simulink model "Control_config"  (R2023b)
settings: Solver=VariableStepAuto  StartTime=0.0  StopTime=inf  RelTol=1e-3
libraries: vrlib x1
settings Model: Creator=angel  LastModifiedBy=angel

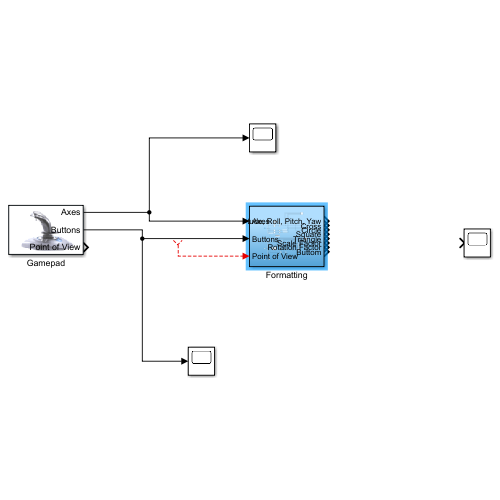
[thumbnail: Simulink's stored preview of the top-level diagram]
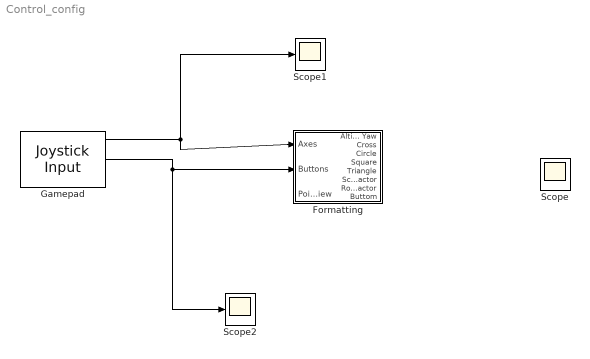
== system Control_config ==
  Formatting : Subsystem
  Gamepad : vrlib/Joystick Input  joyid=1  adjustports=on  forcefeed=off
  Scope : Scope
  Scope1 : Scope
  Scope2 : Scope
  wires:
  Gamepad/2 -> Scope2/1, Formatting/2(Buttons)
  ? -> Formatting/3(Point of View)
  Gamepad/1 -> Scope1/1, Formatting/1(Axes)

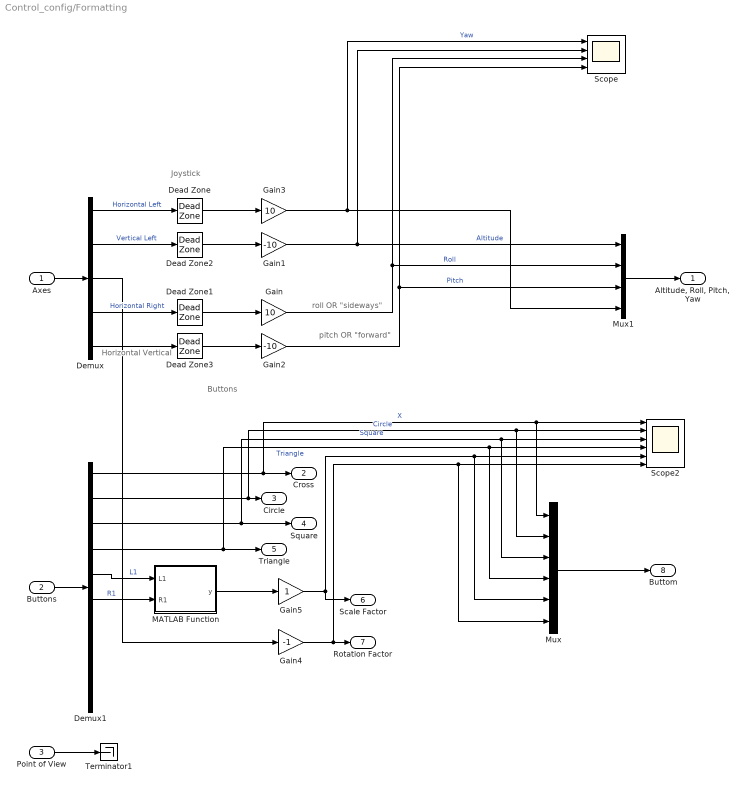
== system Control_config/Formatting ==
  note: Joystick
  note: Horizontal Vertical
  note: roll OR "sideways"
  note: pitch OR "forward"
  note: Buttons
  Axes : Inport
  Buttons : Inport  Port=2
  Point of View : Inport  Port=3
  Dead Zone{,1..3} (4 alike) : DeadZone  LowerValue=-0.2  UpperValue=0.2
  Demux : Demux  Outputs=5
  Demux1 : Demux  Outputs=10
  Gain : Gain  Gain=10
  Gain1 : Gain  Gain=-10
  Gain2 : Gain  Gain=-10
  Gain3 : Gain  Gain=10
  Gain4 : Gain  Gain=-1
  Gain5 : Gain
  MATLAB Function : MATLAB Function  TreatAsAtomicUnit=on
  Mux : Mux  Inputs=6
  Mux1 : Mux
  Scope : Scope  NumInputPorts=4
  Scope2 : Scope  NumInputPorts=6
  Terminator1 : Terminator
  "Altitude, Roll, Pitch, Yaw" : Outport
  Cross : Outport  Port=2
  Circle : Outport  Port=3
  Square : Outport  Port=4
  Triangle : Outport  Port=5
  Scale Factor : Outport  Port=6
  Rotation Factor : Outport  Port=7
  Buttom : Outport  Port=8
  wires:
  Axes/1 -> Demux/1
  Demux/5 -> Dead Zone3/1
  Demux/4 -> Dead Zone1/1  "Horizontal Right"
  Demux/1 -> Dead Zone/1  "Horizontal Left"
  Dead Zone1/1 -> Gain/1
  Demux/2 -> Dead Zone2/1  "Vertical Left"
  Dead Zone2/1 -> Gain1/1
  Dead Zone/1 -> Gain3/1
  Point of View/1 -> Terminator1/1
  Dead Zone3/1 -> Gain2/1
  Gain2/1 -> Scope/4, Mux1/3  "Pitch"
  Gain/1 -> Scope/3, Mux1/2  "Roll"
  Gain3/1 -> Scope/1, Mux1/4  "Yaw"
  Gain1/1 -> Scope/2, Mux1/1  "Altitude"
  Buttons/1 -> Demux1/1
  Demux1/1 -> Mux/1, Scope2/1, Cross/1  "X"
  Demux1/2 -> Scope2/2, Mux/2, Circle/1  "Circle"
  Demux1/3 -> Square/1, Scope2/3, Mux/3  "Square"
  Demux1/4 -> Scope2/4, Mux/4, Triangle/1  "Triangle"
  Demux/3 -> Gain4/1
  Demux1/5 -> MATLAB Function/1(L1)  "L1"
  Gain5/1 -> Scope2/5, Mux/5, Scale Factor/1
  Gain4/1 -> Scope2/6, Mux/6, Rotation Factor/1
  Demux1/6 -> MATLAB Function/2(R1)  "R1"
  MATLAB Function/1(y) -> Gain5/1
  Mux1/1 -> "Altitude, Roll, Pitch, Yaw"/1
  Mux/1 -> Buttom/1

== matlab function Control_config/Formatting/MATLAB Function ==
  data: L1 input; y output; R1 input
function y = fcn(L1, R1)

if L1 == 1 && R1 == 0
    y = -1;
elseif R1 == 1 && L1 == 0
    y = 1;
else
    y = 0;
end

end
